simulink model "Observer_Luenberger_sensibilite_II_2023b"  (R2025a)
settings: Solver=FixedStepAuto  StartTime=0.0  StopTime=Inf  FixedStep=sub_step_size  RelTol=1e-3
PostLoadFcn:
  | , if any(exist('dsrtsu_mdlpostloadfcn', 'file') ~= 0), dsrtsu_mdlpostloadfcn('Execute', bdroot); end,
InitFcn:
  | , if any(exist('rtifpga_mdlclblib', 'file') ~= 0), rtifpga_mdlclblib('Init', bdroot); end,
values from neighbouring files (symbols this model uses):
  grandeurs_modales = load('grandeurs_modales.mat').MODAL    [varDQ_Observateur.m]
  k = 6    [varDQ_Observateur.m]
  mode_init = 1    [varDQ_Observateur.m]
  nb_plaques = numel(grandeurs_modales.n_modes)    [varDQ_Observateur.m]
  plaque_init = 1    [varDQ_Observateur.m]
  step_size = 1/frequency    (= 1.25e-06)    [varDQ_Observateur.m]
  V = 80    [varDQ_Observateur.m]
undefined symbols (not defined in the file or in its folder): conf, DiscIntNeverNeededParam
libraries: simulink x5, eeGeneralControl x2, slpidlib x1
Description:
  | Standard RTI1202 template.
  | Supported MATLAB version:  R2021a.
settings Model: Tag=RTI1202  DSRTSU_INTERNAL_RTI_VER=610  DSRTSU_INTERNAL_RTI_TYPE=rti1202  RTICANMMDATA=struct('GeneralSetupData',struct('modelroot','C:\Users\VM-User\Desktop\MigrationScripts','generalsettings',struct('filesettings',struct('destfolder',struct('Name','RTICANMM_FILES','Check',1),'buildfolder',struct('Name','.','Check',1),'AbsDestfolder',struct('Name','C:\Users\VM-User\Desktop\MigrationScripts\RTICANMM_FILES'),'AbsBuildfolder',struct('Name','C:\Users\VM-User\Desktop\MigrationScripts'))),'options',struct('addpaths',1,'rmpaths',1,'addtrcexclusion',true,'cannavigator',struct('checkmonitoring',0),'show_usrtrc',0,'use_usrtrc',0),'advanced',struct('options',ones(1,100)),'MPSetup',{{}},'RTI',struct('Type','RTI1202','Ver','7.17','Date','02-Nov-2021'),'modelname','','block','untitled'))  DSRTSU_INTERNAL_RTIFPGA=200  DSRTSU_INTERNAL_RTISTBM_VER=22.2  Creator=g.eymard  LastModifiedBy=user
settings SolverCC: AlgebraicLoopSolver=TrustRegion
settings DataIOCC: ReturnWorkspaceOutputs=off
settings OptimizationCC: BlockReduction=off  OptimizeBlockIOStorage=off  BufferReuse=off  GlobalBufferReuse=off  ExpressionFolding=off  LocalBlockOutputs=off  OptimizeDataStoreBuffers=off  BusAssignmentInplaceUpdate=off
settings DebuggingCC: UnconnectedInputMsg=warning  UnconnectedOutputMsg=warning  UnconnectedLineMsg=warning  PregeneratedLibrarySubsystemCodeDiagnostic=none  ArithmeticOperatorsInVariantConditions=warning
settings HardwareCC: ProdBitPerPointer=32.0  ProdBitPerSizeT=32.0  ProdBitPerPtrDiffT=32.0  ProdLargestAtomicInteger=Integer  ProdEndianess=BigEndian  ProdWordSize=32.0  ProdLongLongMode=on  ProdHWDeviceType=Custom Processor->Custom  TargetIntDivRoundTo=Zero  TargetEndianess=BigEndian  TargetHWDeviceType=Custom Processor->Custom
settings ModelReferenceCC: EnableRefExpFcnMdlSchedulingChecks=on  EnableParallelModelReferenceBuilds=on  ParallelModelReferenceMATLABWorkerInit=Load Top Model
settings SFSimCC: SimUseLocalCustomCode=off  MATLABDynamicMemAlloc=off  CustomCodeUndefinedFunction=UseInterfaceOnly
settings RTWCC: SystemTargetFile=rti1202.tlc  MakeCommand=make_rti  TemplateMakefile=rti1202.tmf  RTWUseLocalCustomCode=off  GPUComputeCapability=3.5  DLArmComputeVersion=19.05  Description=dSPACE DS1202 Hardware Platform
settings CodeAppCC: StateflowObjectComments=on
settings STFCustomTargetCC: SystemTargetFile=rti1202.tlc  MultiwordLength=2048.0  DynamicStringBufferSize=256.0  ParMdlRefBuildCompliant=on  GRTInterface=off  TaskMode=Low jitter, low latency tasks  FSIValue=0  TRCIsOmitVdOn=off  NISValue=1  LoadApplNonUI=ON  TRCGenerateDerivatives=off  RTICfgSetVer=610.0  PlatformSelectionPopup=Platform Name  CCompilerOptimizationOptsPopup_=Default  TimeScaleFactor=1.0  BoardName=ds1202  CCompilerOptimizationOptsNonUI=USE_DEFAULT  ExecutionMode=real-time  BoardNameNonUI=ds1202  EnableRealTimeTesting=on  InitialSimState=RUN  AllowReservedHostServiceNums=off  ExecutionModeNonUI=RTSIM  LoadAfterBuild=on  NetworkClientNonUI=OPTION_DISABLED  EnableRealTimeTestingNonUI=ON  TimeScaleFactorNonUI=OPTION_DISABLED  LoadToFlash=off  VDFType=TRC  TRCGenerateVirtualBlocks=off  TRCOnlyGlobals=off  TaskModeNonUI=LOW_JITTER  AssertionMode=OFF  TRCGenerateParamValues=off  TRCGenerateLabels=off  TRCGenerateStates=off
settings GRTTargetCC: TargetLangStandard=C89/C90 (ANSI)  CompOptLevelCompliant=off  ConcurrentExecutionCompliant=off  CombineOutputUpdateFcns=off  MatFileLogging=off  CPPClassGenCompliant=off  UseToolchainInfoCompliant=off
settings ConfigComp: CovMetricSettings=dswe

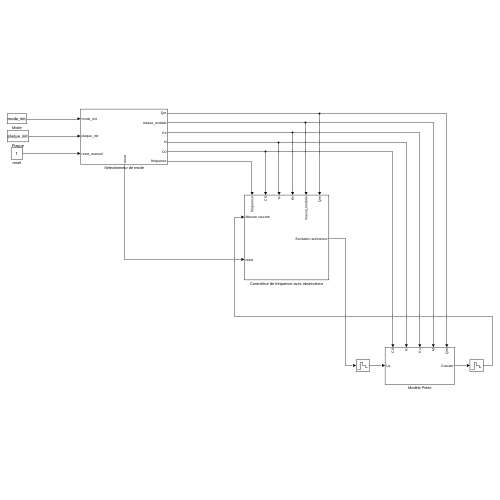
[thumbnail: Simulink's stored preview of the top-level diagram]
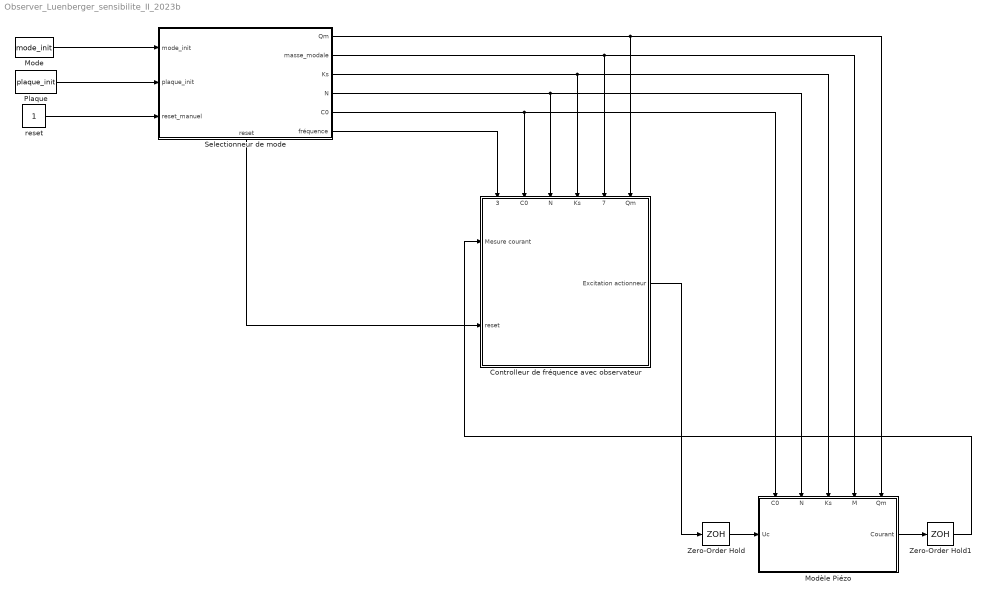
== system Observer_Luenberger_sensibilite_II_2023b ==
  Controlleur de fréquence avec observateur : Subsystem
      settings: PortSchema="{\"entries\":[{\"content\":{\"sides\":[{\"content\":{\"connectorIds\":[\"In1\",\"In2\"]},\"type\":\"ConnectorPlacement.EquallySpacedRectSide\",\"uuid\":\"530a0f3e-ee2a-4c6d-8269-1953a5690c3e\"},{\"content\":{\"connectorIds\":[\"Out1\"],\"side\":\"RIGHT\"},\"type\":\"ConnectorPlacement.EquallySpacedRectSide\",\"uuid\":\"d68bd64f-59c0-41d5-a325-75bb2cb6ca14\"},{\"content\":{\"connectorIds\":[\"In3\",\"In4\",\"In5\",\"In6\",\"In7\",\"In8\"],\"side\":\"TOP\"},\"type\":\"ConnectorPlacement.EquallySpacedRectSide\",\"uuid\":\"5a147631-f81e-4841-8249-4b54ec8a3c6f\"}]},\"type\":\"ConnectorPlacement.EquallySpacedConnector\",\"uuid\":\"7e21fd24-4eb3-483e-b19b-d5a2d9cc9389\"}],\"packageUris\":[\"http://schema.mathworks.com/mf0/Connector/R2020b\"],\"version\":\"1.0\"}"
  Mode : Constant  Value=mode_init  SampleTime=step_size
  Modèle Piézo : Subsystem
      settings: PortSchema="{\"entries\":[{\"content\":{\"sides\":[{\"content\":{\"connectorIds\":[\"In1\"]},\"type\":\"ConnectorPlacement.EquallySpacedRectSide\",\"uuid\":\"faf53970-2953-4ceb-88b4-68bddd4a0fc8\"},{\"content\":{\"connectorIds\":[\"Out1\"],\"side\":\"RIGHT\"},\"type\":\"ConnectorPlacement.EquallySpacedRectSide\",\"uuid\":\"a2d81363-6c92-409a-946a-c9fbc60f8e0e\"},{\"content\":{\"connectorIds\":[\"In2\",\"In3\",\"In4\",\"In5\",\"In6\"],\"side\":\"TOP\"},\"type\":\"ConnectorPlacement.EquallySpacedRectSide\",\"uuid\":\"99e0e8a0-eb56-42eb-b6d4-0f3431f01427\"}]},\"type\":\"ConnectorPlacement.EquallySpacedConnector\",\"uuid\":\"f1fccc4c-7076-4c73-816a-62f4c7feacf8\"}],\"packageUris\":[\"http://schema.mathworks.com/mf0/Connector/R2020b\"],\"version\":\"1.0\"}"
  Plaque : Constant  Value=plaque_init  SampleTime=step_size
  Selectionneur de mode : Subsystem
      settings: PortSchema="{\"entries\":[{\"content\":{\"sides\":[{\"content\":{\"connectorIds\":[\"In1\",\"In2\",\"In3\"]},\"type\":\"ConnectorPlacement.EquallySpacedRectSide\",\"uuid\":\"d44dafbb-4531-4740-8f88-9444e013c349\"},{\"content\":{\"connectorIds\":[\"Out1\",\"Out2\",\"Out3\",\"Out4\",\"Out5\",\"Out6\"],\"side\":\"RIGHT\"},\"type\":\"ConnectorPlacement.EquallySpacedRectSide\",\"uuid\":\"a0382d4c-1f36-46aa-81e2-f668b2a7eaab\"},{\"content\":{\"side\":\"TOP\"},\"type\":\"ConnectorPlacement.EquallySpacedRectSide\",\"uuid\":\"83c5ddd4-1965-4675-8f4e-255b2976aa40\"},{\"content\":{\"connectorIds\":[\"Out7\"],\"side\":\"BOTTOM\"},\"type\":\"ConnectorPlacement.EquallySpacedRectSide\",\"uuid\":\"40dab04f-efa3-4035-a07f-cd814a6077f4\"}]},\"type\":\"ConnectorPlacement.EquallySpacedConnector\",\"uuid\":\"ca871b34-0c20-4adb-897c-f336d60f682d\"}],\"packageUris\":[\"http://schema.mathworks.com/mf0/Connector/R2020b\"],\"version\":\"1.0\"}"
  Zero-Order Hold : ZeroOrderHold  SampleTime=step_size
  Zero-Order Hold1 : ZeroOrderHold  SampleTime=step_size
  reset : Constant  SampleTime=step_size
  wires:
  Mode/1 -> Selectionneur de mode/1(mode_init)
  Plaque/1 -> Selectionneur de mode/2(plaque_init)
  reset/1 -> Selectionneur de mode/3(reset_manuel)
  Selectionneur de mode/7(reset) -> Controlleur de fréquence avec observateur/2(reset)
  Selectionneur de mode/6(fréquence) -> Controlleur de fréquence avec observateur/3(fréquence)
  Selectionneur de mode/5(C0) -> Modèle Piézo/2(C0), Controlleur de fréquence avec observateur/4(C0)
  Selectionneur de mode/2(masse_modale) -> Modèle Piézo/5(M), Controlleur de fréquence avec observateur/7(masse_modale)
  Selectionneur de mode/4(N) -> Modèle Piézo/3(N), Controlleur de fréquence avec observateur/5(N)
  Selectionneur de mode/3(Ks) -> Modèle Piézo/4(Ks), Controlleur de fréquence avec observateur/6(Ks)
  Controlleur de fréquence avec observateur/1(Excitation actionneur) -> Zero-Order Hold/1
  Modèle Piézo/1(Courant) -> Zero-Order Hold1/1
  Zero-Order Hold/1 -> Modèle Piézo/1(Uc)
  Zero-Order Hold1/1 -> Controlleur de fréquence avec observateur/1(Mesure courant)
  Selectionneur de mode/1(Qm) -> Modèle Piézo/6(Qm), Controlleur de fréquence avec observateur/8(Qm)

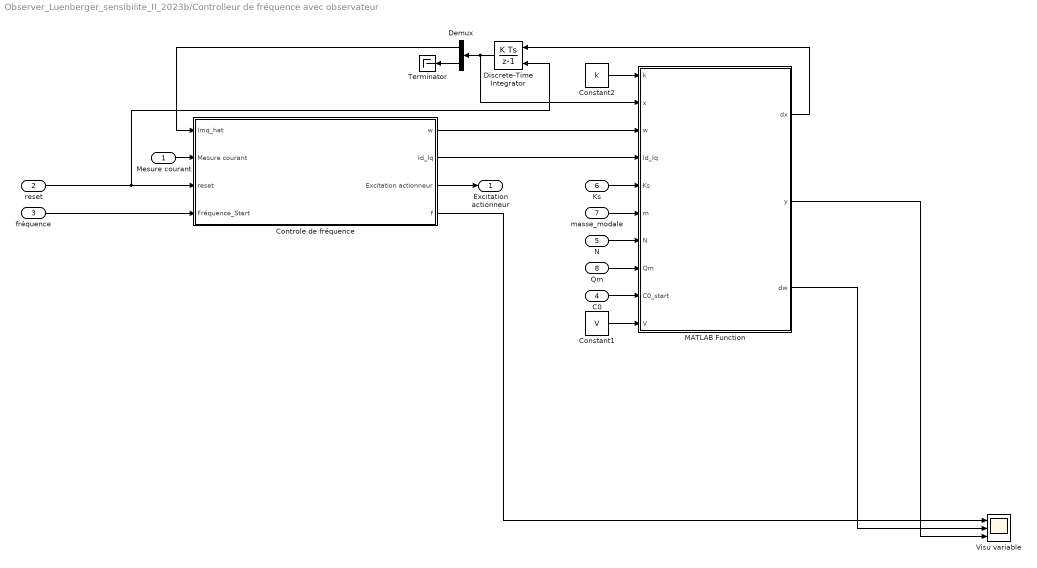
== system Observer_Luenberger_sensibilite_II_2023b/Controlleur de fréquence avec observateur ==
  Mesure courant : Inport
  reset : Inport  Port=2
  fréquence : Inport  Port=3
  C0 : Inport  Port=4
  N : Inport  Port=5
  Ks : Inport  Port=6
  masse_modale : Inport  Port=7
  Qm : Inport  Port=8
  Constant1 : Constant  Value=V  SampleTime=step_size
  Constant2 : Constant  Value=k  SampleTime=step_size
  Controle de fréquence : Subsystem
  Demux : Demux  Outputs=2
  Discrete-Time Integrator : DiscreteIntegrator  ExternalReset=rising  InitialCondition=[0; 0]  SampleTime=-1  ICPrevOutput=DiscIntNeverNeededParam  ICPrevScaledInput=DiscIntNeverNeededParam
  MATLAB Function : MATLAB Function  TreatAsAtomicUnit=on
  Terminator : Terminator
  Visu variable : Scope  NumInputPorts=3
      settings: ActiveDisplayYMinimum=-632.5898  ActiveDisplayYMaximum=4274.0061
  Excitation actionneur : Outport
  wires:
  Controle de fréquence/2(Id_Iq) -> MATLAB Function/4(Id_Iq)
  Discrete-Time Integrator/1 -> MATLAB Function/2(x), Demux/1
  Mesure courant/1 -> Controle de fréquence/2(Mesure courant)
  Controle de fréquence/1(w) -> MATLAB Function/3(w)
  Controle de fréquence/3(Excitation actionneur) -> Excitation actionneur/1
  MATLAB Function/1(dx) -> Discrete-Time Integrator/1
  Demux/1 -> Controle de fréquence/1(Imq_hat)
  Controle de fréquence/4(f) -> Visu variable/1
  MATLAB Function/3(dw) -> Visu variable/2
  MATLAB Function/2(y) -> Visu variable/3
  reset/1 -> Discrete-Time Integrator/2, Controle de fréquence/3(reset)
  Demux/2 -> Terminator/1
  fréquence/1 -> Controle de fréquence/4(Fréquence_Start)
  masse_modale/1 -> MATLAB Function/6(m)
  Ks/1 -> MATLAB Function/5(Ks)
  N/1 -> MATLAB Function/7(N)
  Constant1/1 -> MATLAB Function/10(V)
  C0/1 -> MATLAB Function/9(C0_start)
  Qm/1 -> MATLAB Function/8(Qm)
  Constant2/1 -> MATLAB Function/1(k)

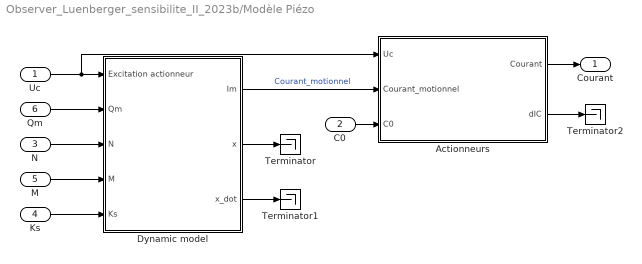
== system Observer_Luenberger_sensibilite_II_2023b/Modèle Piézo ==
  Uc : Inport
  C0 : Inport  Port=2
  N : Inport  Port=3
  Ks : Inport  Port=4
  M : Inport  Port=5
  Qm : Inport  Port=6
  Actionneurs : Subsystem
  Dynamic model : Subsystem
  Terminator : Terminator
  Terminator1 : Terminator
  Terminator2 : Terminator
  Courant : Outport
  wires:
  Actionneurs/2(dIC) -> Terminator2/1
  Dynamic model/3(x_dot) -> Terminator1/1
  Dynamic model/2(x) -> Terminator/1
  Dynamic model/1(Im) -> Actionneurs/2(Courant_motionnel)  "Courant_motionnel"
  M/1 -> Dynamic model/4(M)
  N/1 -> Dynamic model/3(N)
  Ks/1 -> Dynamic model/5(Ks)
  Uc/1 -> Actionneurs/1(Uc), Dynamic model/1(Excitation actionneur)
  Actionneurs/1(Courant) -> Courant/1
  C0/1 -> Actionneurs/3(C0)
  Qm/1 -> Dynamic model/2(Qm)

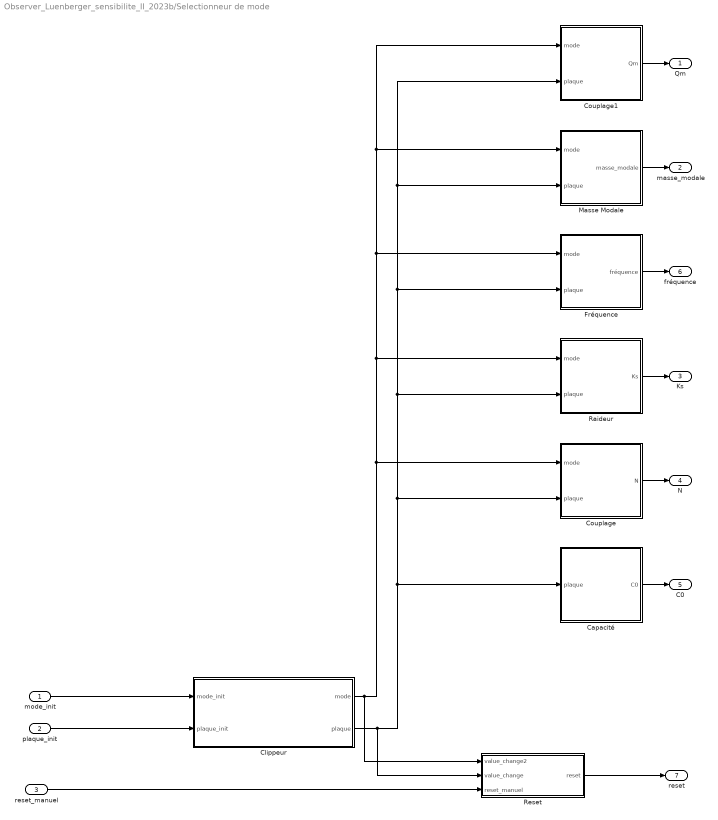
== system Observer_Luenberger_sensibilite_II_2023b/Selectionneur de mode ==
  mode_init : Inport
  plaque_init : Inport  Port=2
  reset_manuel : Inport  Port=3
  Capacité : Subsystem
  Clippeur : Subsystem
  Couplage : Subsystem
  Couplage1 : Subsystem
  Fréquence : Subsystem
  Masse Modale : Subsystem
  Raideur : Subsystem
  Reset : Subsystem
  Qm : Outport
  masse_modale : Outport  Port=2
  Ks : Outport  Port=3
  N : Outport  Port=4
  C0 : Outport  Port=5
  fréquence : Outport  Port=6
  reset : Outport  Port=7
  wires:
  mode_init/1 -> Clippeur/1(mode_init)
  Masse Modale/1(masse_modale) -> masse_modale/1
  Reset/1(reset) -> reset/1
  plaque_init/1 -> Clippeur/2(plaque_init)
  Fréquence/1(fréquence) -> fréquence/1
  reset_manuel/1 -> Reset/3(reset_manuel)
  Raideur/1(Ks) -> Ks/1
  Couplage/1(N) -> N/1
  Capacité/1(C0) -> C0/1
  Clippeur/1(mode) -> Reset/1(value_change2), Couplage/1(mode), Fréquence/1(mode), Couplage1/1(mode), Masse Modale/1(mode), Raideur/1(mode)
  Clippeur/2(plaque) -> Reset/2(value_change), Capacité/1(plaque), Couplage/2(plaque), Fréquence/2(plaque), Couplage1/2(plaque), Masse Modale/2(plaque), Raideur/2(plaque)
  Couplage1/1(Qm) -> Qm/1

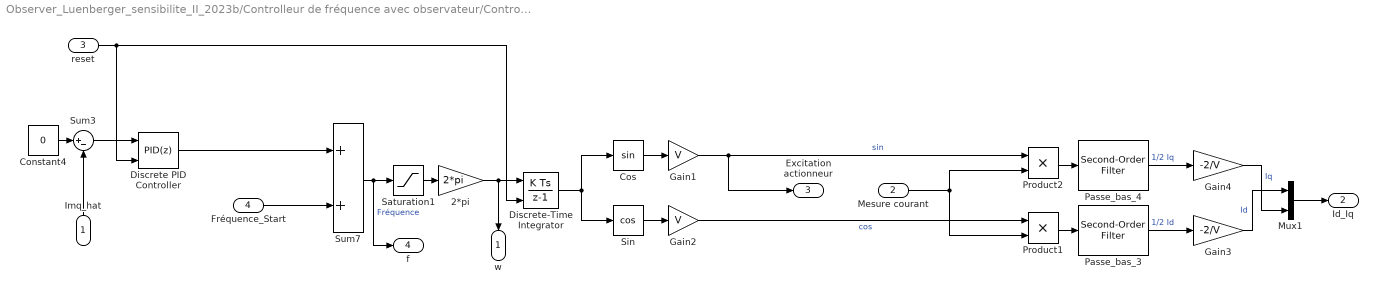
== system Observer_Luenberger_sensibilite_II_2023b/Controlleur de fréquence avec observateur/Controle de fréquence ==
  Imq_hat : Inport
  Mesure courant : Inport  Port=2
  reset : Inport  Port=3
  Fréquence_Start : Inport  Port=4
  " Mux1" : Mux  Inputs=2
  2*pi : Gain  Gain=2*pi
  Constant4 : Constant  Value=0  SampleTime=step_size
  Cos : Trigonometry
  Discrete PID Controller : slpidlib/PID Controller  Controller=PID  Form=Parallel  TimeDomain=Discrete-time  UseExternalTs=off  SampleTime=step_size  IntegratorMethod=Forward Euler  FilterMethod=Forward Euler  ControllerParametersSource=internal  P=-10000  I=-9e6/2  UseKiTs=off  D=0  UseExternalDerivativeSource=off  N=100  UseFilter=on  TunerSelectOption=Transfer Function Based (PID Tuner App)  InitialConditionSource=internal  InitialConditionForIntegrator=0  InitialConditionForFilter=0  DifferentiatorICPrevScaledInput=0  ExternalReset=rising  TrackingMode=off  Kt=1  LimitOutput=off  SatLimitsSource=internal  UpperSaturationLimit=inf  LowerSaturationLimit=-inf  LinearizeAsGain=off  AntiWindupMode=none  Kb=1  LimitIntegrator=off  UpperIntegratorSaturationLimit=inf  LowerIntegratorSaturationLimit=-inf  POutMin=[]  POutMax=[]  IOutMin=[]  IOutMax=[]  DOutMin=[]  DOutMax=[]  NOutMin=[]  NOutMax=[]  SumOutMin=[]  SumOutMax=[]  SaturationOutMin=[]  SaturationOutMax=[]  PParamMin=[]  PParamMax=[]  IParamMin=[]  IParamMax=[]  DParamMin=[]  DParamMax=[]  NParamMin=[]  NParamMax=[]  KbParamMin=[]  KbParamMax=[]  KtParamMin=[]  KtParamMax=[]  KbOutMin=[]  KbOutMax=[]  KtOutMin=[]  KtOutMax=[]  IntegratorOutMin=[]  IntegratorOutMax=[]  FilterOutMin=[]  FilterOutMax=[]  SumI1OutMin=[]  SumI1OutMax=[]  SumI2OutMin=[]  SumI2OutMax=[]  SumI3OutMin=[]  SumI3OutMax=[]  SumI4OutMin=[]  SumI4OutMax=[]  SumDOutMin=[]  SumDOutMax=[]  DifferentiatorOutMin=[]  DifferentiatorOutMax=[]  FilterDiffOutCoefMin=[]  FilterDiffOutCoefMax=[]  ReciprocalOutMin=[]  ReciprocalOutMax=[]  SumDenOutMin=[]  SumDenOutMax=[]  SumNumOutMin=[]  SumNumOutMax=[]  DivideOutMin=[]  DivideOutMax=[]  UdiffTsProdOutMin=[]  UdiffTsProdOutMax=[]  NTsProdOutMin=[]  NTsProdOutMax=[]  UintegralTsProdOutMin=[]  UintegralTsProdOutMax=[]  UngainTsProdOutMin=[]  UngainTsProdOutMax=[]  ClampingZeroOutDataTypeStr=Inherit: Inherit via back propagation  ClampingZeroOutMin=[]  ClampingZeroOutMax=[]  FilterDenConstantOutDataTypeStr=Inherit: Inherit via back propagation  FilterDenConstantOutMin=[]  FilterDenConstantOutMax=[]  PCopyOutDataTypeStr=Inherit: Inherit via back propagation  PCopyOutMin=[]  PCopyOutMax=[]  NCopyOutDataTypeStr=Inherit: Inherit via back propagation  NCopyOutMin=[]  NCopyOutMax=[]  IntegratorContinuousStateAttributes=''  IntegratorStateMustResolveToSignalObject=off  IntegratorRTWStateStorageClass=Auto  FilterContinuousStateAttributes=''  FilterStateMustResolveToSignalObject=off  FilterRTWStateStorageClass=Auto  ParallelPVariant=InternalParameters  IdealPVariant=Disabled  IVariant=InternalParameters  DVariant=InternalParameters  IntegratorVariant=Discrete  SatVariant=Disabled  AWVariant=Passthrough  PCopyVariant=Disabled  TRVariant=Disabled  FdbkBlocksVariant=Forward  IdealPFdbkVariant=Disabled  SatFdbkVariant=Disabled  DerivativeFilterVariant=ForwardEulerFilter  NVariant=InternalParameters  NCopyVariant=Disabled  FilterICVariant=InternalICsFilter  IntegratorICVariant=InternalICs  ExternalResetVariant=ExternalReset  TRSumVariant=Passthrough  SumFdbkVariant=Disabled  SumVariant=Sum_PID  TsampFilterVariant=InternalTs  TsampNgainVariant=Passthrough  TsampIntegralVariant=Disabled_SignalSpec  ExternalSaturationOutDataTypeStr=Inherit: Same as second input  DerivativeSourceVariant=ErrorSignal  PreIntVariant=InternalPreInt
  Discrete-Time Integrator : DiscreteIntegrator  ExternalReset=rising  SampleTime=-1  ICPrevOutput=DiscIntNeverNeededParam  ICPrevScaledInput=DiscIntNeverNeededParam
  Gain1 : Gain  Gain=V
  Gain2 : Gain  Gain=V
  Gain3 : Gain  Gain=-2/V
  Gain4 : Gain  Gain=-2/V
  Passe_bas_3 : eeGeneralControl/Second-Order Filter  FilterType=Low-pass  fn=50  Zeta=0.707  Ts=-1  A0=1e-6  Ph0=0  f0=0  b0=0
  Passe_bas_4 : eeGeneralControl/Second-Order Filter  FilterType=Low-pass  fn=50  Zeta=0.707  Ts=-1  A0=1e-6  Ph0=0  f0=0  b0=0
  Product1 : Product
  Product2 : Product
  Saturation1 : Saturate  UpperLimit=inf  LowerLimit=0
  Sin : Trigonometry  Operator=cos
  Sum3 : Sum  Inputs=|+-
  Sum7 : Sum
  w : Outport
  Id_Iq : Outport  Port=2
  Excitation actionneur : Outport  Port=3
  f : Outport  Port=4
  wires:
  Cos/1 -> Gain1/1
  Fréquence_Start/1 -> Sum7/2
  Discrete-Time Integrator/1 -> Sin/1, Cos/1
  2*pi/1 -> Discrete-Time Integrator/1, w/1
  Sin/1 -> Gain2/1
  Discrete PID Controller/1 -> Sum7/1
  Constant4/1 -> Sum3/1
  Imq_hat/1 -> Sum3/2
  Sum3/1 -> Discrete PID Controller/1
  Gain2/1 -> Product1/1  "cos"
  Passe_bas_3/1 -> Gain3/1  "1/2 Id"
  Mesure courant/1 -> Product2/2, Product1/2
  Product2/1 -> Passe_bas_4/1
  Passe_bas_4/1 -> Gain4/1  "1/2 Iq"
  Product1/1 -> Passe_bas_3/1
  Gain1/1 -> Excitation actionneur/1, Product2/1  "sin"
  " Mux1"/1 -> Id_Iq/1
  Sum7/1 -> f/1, Saturation1/1  "Fréquence"
  Saturation1/1 -> 2*pi/1
  reset/1 -> Discrete-Time Integrator/2, Discrete PID Controller/2
  Gain4/1 -> " Mux1"/2  "Iq"
  Gain3/1 -> " Mux1"/1  "Id"

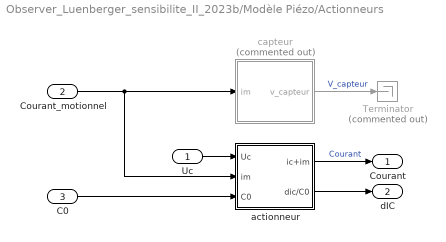
== system Observer_Luenberger_sensibilite_II_2023b/Modèle Piézo/Actionneurs ==
  Uc : Inport
  Courant_motionnel : Inport  Port=2
  C0 : Inport  Port=3
  Terminator : Terminator  Commented=on
  actionneur : Subsystem
  capteur : Subsystem  Commented=on
  Courant : Outport
  dIC : Outport  Port=2
  wires:
  actionneur/1(ic+im) -> Courant/1  "Courant"
  Uc/1 -> actionneur/1(Uc)
  capteur/1(v_capteur) -> Terminator/1  "V_capteur"
  Courant_motionnel/1 -> capteur/1(im), actionneur/2(im)
  actionneur/2(dic/C0) -> dIC/1
  C0/1 -> actionneur/3(C0)

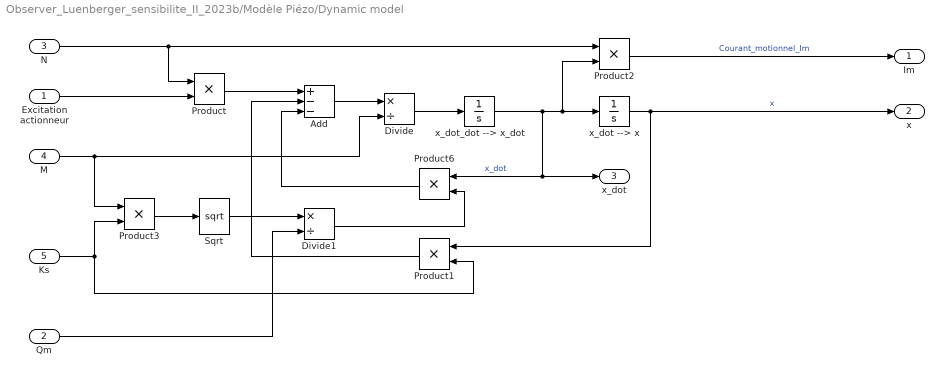
== system Observer_Luenberger_sensibilite_II_2023b/Modèle Piézo/Dynamic model ==
  Excitation actionneur : Inport
  Qm : Inport  Port=2
  N : Inport  Port=3
  M : Inport  Port=4
  Ks : Inport  Port=5
  Add : Sum  Inputs=+--
  Divide : Product  Inputs=*/
  Divide1 : Product  Inputs=*/
  Product{,1..3,6} (5 alike) : Product
  Sqrt : Sqrt
  x_dot --> x : Integrator
  x_dot_dot --> x_dot : Integrator
  Im : Outport
  x : Outport  Port=2
  x_dot : Outport  Port=3
  wires:
  M/1 -> Divide/2, Product3/1
  N/1 -> Product/1, Product2/1
  x_dot_dot --> x_dot/1 -> Product2/2, x_dot --> x/1, x_dot/1, Product6/1  "x_dot"
  Ks/1 -> Product1/2, Product3/2
  Product1/1 -> Add/2
  Divide1/1 -> Product6/2
  Product6/1 -> Add/3
  x_dot --> x/1 -> x/1, Product1/1  "x"
  Add/1 -> Divide/1
  Product3/1 -> Sqrt/1
  Product/1 -> Add/1
  Excitation actionneur/1 -> Product/2
  Divide/1 -> x_dot_dot --> x_dot/1
  Product2/1 -> Im/1  "Courant_motionnel_Im"
  Sqrt/1 -> Divide1/1
  Qm/1 -> Divide1/2

== system Observer_Luenberger_sensibilite_II_2023b/Selectionneur de mode/Capacité ==
  plaque : Inport
  Constant1 : Constant  Value=grandeurs_modales.C0  SampleTime=step_size
  Selector : Selector  InputPortWidth=nb_plaques  IndexOptions=Index vector (port)  Indices=[1 3]  OutputSizes=1
  C0 : Outport
  wires:
  Constant1/1 -> Selector/1
  Selector/1 -> C0/1
  plaque/1 -> Selector/2

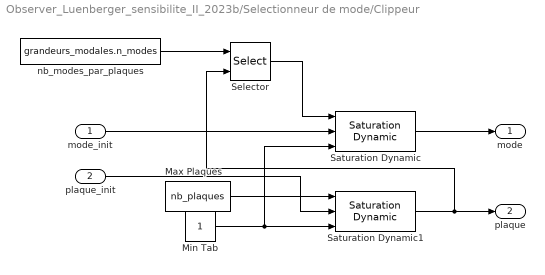
== system Observer_Luenberger_sensibilite_II_2023b/Selectionneur de mode/Clippeur ==
  mode_init : Inport
  plaque_init : Inport  Port=2
  Max Plaques : Constant  Value=nb_plaques  SampleTime=step_size
  Min Tab : Constant  SampleTime=step_size
  Saturation Dynamic : simulink/Discontinuities/Saturation Dynamic  OutMin=[]  OutMax=[]  OutDataTypeStr=Inherit: Same as second input  OutDataType=fixdt(1, 16)  OutScaling=2^-10  DoSatur=off
  Saturation Dynamic1 : simulink/Discontinuities/Saturation Dynamic  OutMin=[]  OutMax=[]  OutDataTypeStr=Inherit: Same as second input  OutDataType=fixdt(1, 16)  OutScaling=2^-10  DoSatur=off
  Selector : Selector  InputPortWidth=nb_plaques  IndexOptions=Index vector (port)  Indices=[1 3]  OutputSizes=1
  nb_modes_par_plaques : Constant  Value=grandeurs_modales.n_modes  SampleTime=step_size
  mode : Outport
  plaque : Outport  Port=2
  wires:
  Min Tab/1 -> Saturation Dynamic/3, Saturation Dynamic1/3
  Saturation Dynamic1/1 -> plaque/1, Selector/2
  plaque_init/1 -> Saturation Dynamic1/2
  Max Plaques/1 -> Saturation Dynamic1/1
  nb_modes_par_plaques/1 -> Selector/1
  Saturation Dynamic/1 -> mode/1
  Selector/1 -> Saturation Dynamic/1
  mode_init/1 -> Saturation Dynamic/2

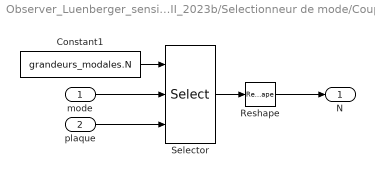
== system Observer_Luenberger_sensibilite_II_2023b/Selectionneur de mode/Couplage ==
  mode : Inport
  plaque : Inport  Port=2
  Constant1 : Constant  Value=grandeurs_modales.N  SampleTime=step_size
  Reshape : Reshape  OutputDimensionality=Customize  OutputDimensions=1
  Selector : Selector  NumberOfDimensions=2  InputPortWidth=3  IndexOptions=Index vector (port),Index vector (port)  Indices=[1 3],1  OutputSizes=1,1
  N : Outport
  wires:
  Constant1/1 -> Selector/1
  mode/1 -> Selector/2
  Selector/1 -> Reshape/1
  plaque/1 -> Selector/3
  Reshape/1 -> N/1

== system Observer_Luenberger_sensibilite_II_2023b/Selectionneur de mode/Couplage1 ==
  mode : Inport
  plaque : Inport  Port=2
  Constant1 : Constant  Value=grandeurs_modales.Qm  SampleTime=step_size
  Reshape : Reshape  OutputDimensionality=Customize  OutputDimensions=1
  Selector : Selector  NumberOfDimensions=2  InputPortWidth=3  IndexOptions=Index vector (port),Index vector (port)  Indices=[1 3],1  OutputSizes=1,1
  Qm : Outport
  wires:
  Constant1/1 -> Selector/1
  mode/1 -> Selector/2
  Selector/1 -> Reshape/1
  plaque/1 -> Selector/3
  Reshape/1 -> Qm/1

== system Observer_Luenberger_sensibilite_II_2023b/Selectionneur de mode/Fréquence ==
  mode : Inport
  plaque : Inport  Port=2
  Constant1 : Constant  Value=grandeurs_modales.f  SampleTime=step_size
  Reshape : Reshape  OutputDimensionality=Customize  OutputDimensions=1
  Selector : Selector  NumberOfDimensions=2  InputPortWidth=3  IndexOptions=Index vector (port),Index vector (port)  Indices=[1 3],1  OutputSizes=1,1
  fréquence : Outport
  wires:
  Constant1/1 -> Selector/1
  mode/1 -> Selector/2
  Selector/1 -> Reshape/1
  plaque/1 -> Selector/3
  Reshape/1 -> fréquence/1

== system Observer_Luenberger_sensibilite_II_2023b/Selectionneur de mode/Masse Modale ==
  mode : Inport
  plaque : Inport  Port=2
  Constant1 : Constant  Value=grandeurs_modales.M  SampleTime=step_size
  Reshape : Reshape  OutputDimensionality=Customize  OutputDimensions=1
  Selector : Selector  NumberOfDimensions=2  InputPortWidth=3  IndexOptions=Index vector (port),Index vector (port)  Indices=[1 3],1  OutputSizes=1,1
  masse_modale : Outport
  wires:
  Constant1/1 -> Selector/1
  mode/1 -> Selector/2
  plaque/1 -> Selector/3
  Selector/1 -> Reshape/1
  Reshape/1 -> masse_modale/1

== system Observer_Luenberger_sensibilite_II_2023b/Selectionneur de mode/Raideur ==
  mode : Inport
  plaque : Inport  Port=2
  Constant1 : Constant  Value=grandeurs_modales.Ks  SampleTime=step_size
  Reshape : Reshape  OutputDimensionality=Customize  OutputDimensions=1
  Selector : Selector  NumberOfDimensions=2  InputPortWidth=3  IndexOptions=Index vector (port),Index vector (port)  Indices=[1 3],1  OutputSizes=1,1
  Ks : Outport
  wires:
  Constant1/1 -> Selector/1
  mode/1 -> Selector/2
  Selector/1 -> Reshape/1
  plaque/1 -> Selector/3
  Reshape/1 -> Ks/1

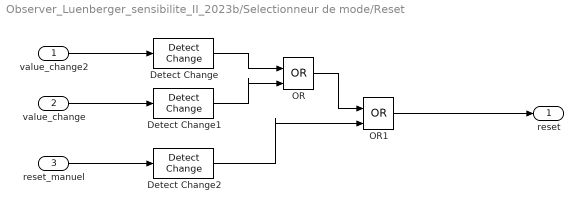
== system Observer_Luenberger_sensibilite_II_2023b/Selectionneur de mode/Reset ==
  value_change2 : Inport
  value_change : Inport  Port=2
  reset_manuel : Inport  Port=3
  Detect Change : simulink/Logic and Bit Operations/Detect Change  vinit=0  OutDataTypeStr=boolean
  Detect Change1 : simulink/Logic and Bit Operations/Detect Change  vinit=0  OutDataTypeStr=boolean
  Detect Change2 : simulink/Logic and Bit Operations/Detect Change  vinit=0  OutDataTypeStr=boolean
  OR : Logic  Operator=OR  IconShape=distinctive  AllPortsSameDT=off  OutDataTypeStr=boolean
  OR1 : Logic  Operator=OR  IconShape=distinctive  AllPortsSameDT=off  OutDataTypeStr=boolean
  reset : Outport
  wires:
  OR1/1 -> reset/1
  Detect Change1/1 -> OR/2
  OR/1 -> OR1/1
  reset_manuel/1 -> Detect Change2/1
  Detect Change/1 -> OR/1
  Detect Change2/1 -> OR1/2
  value_change/1 -> Detect Change1/1
  value_change2/1 -> Detect Change/1

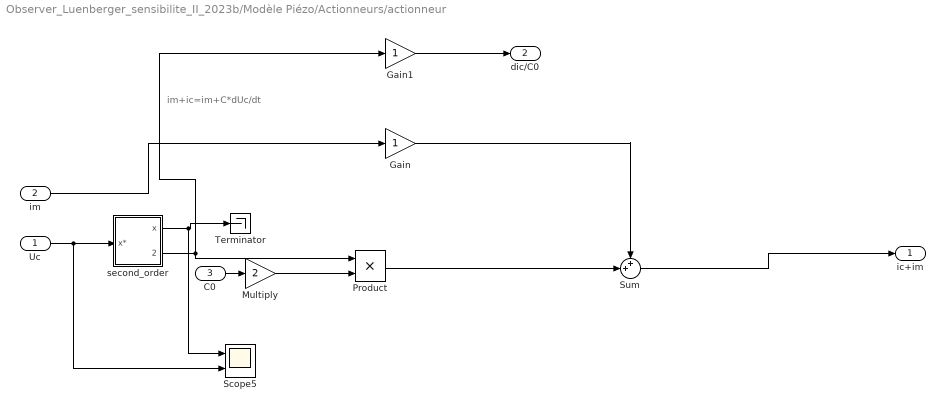
== system Observer_Luenberger_sensibilite_II_2023b/Modèle Piézo/Actionneurs/actionneur ==
  note: im+ic=im+C*dUc/dt
  Uc : Inport
  im : Inport  Port=2
  C0 : Inport  Port=3
  Gain : Gain
  Gain1 : Gain
  Multiply : Gain  Gain=2
  Product : Product
  Scope5 : Scope  NumInputPorts=2
      settings: ActiveDisplayYMinimum=-35.929000784188318  ActiveDisplayYMaximum=42.033035268061695  DataLoggingVariableName=ScopeData5
  Sum : Sum  Inputs=++|
  Terminator : Terminator
  second_order : Subsystem  mask{w=2*pi*50000, m=1}
      mask prompts: w "Pulsation propre"; m "Amortissement"
  ic+im : Outport
  dic/C0 : Outport  Port=2
  wires:
  im/1 -> Gain/1
  Product/1 -> Sum/2
  Sum/1 -> ic+im/1
  Uc/1 -> Scope5/2, second_order/1(x*)
  second_order/2(dx_dt) -> Product/1, Gain1/1
  second_order/1(x) -> Scope5/1, Terminator/1
  Gain/1 -> Sum/1
  Gain1/1 -> dic/C0/1
  Multiply/1 -> Product/2
  C0/1 -> Multiply/1

== system Observer_Luenberger_sensibilite_II_2023b/Modèle Piézo/Actionneurs/capteur ==
  im : Inport
  Add1 : Sum  Inputs=-+
  Gain1 : Gain  Gain=1/conf.det.Ccapt
  Gain2 : Gain  Gain=1/conf.det.Rcapt
  Integrator2 : Integrator
  v_capteur : Outport
  wires:
  Gain2/1 -> Add1/1
  Add1/1 -> Gain1/1
  Gain1/1 -> Integrator2/1  "duc/dt"
  Integrator2/1 -> v_capteur/1, Gain2/1  "v_capteur"
  im/1 -> Add1/2

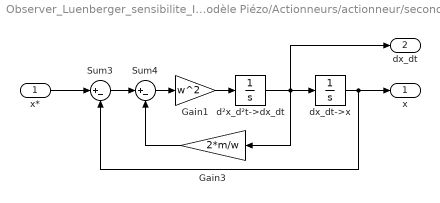
== system Observer_Luenberger_sensibilite_II_2023b/Modèle Piézo/Actionneurs/actionneur/second_order ==
  x* : Inport
  Gain1 : Gain  Gain=w^2
  Gain3 : Gain  Gain=2*m/w
  Sum3 : Sum  Inputs=|+-
  Sum4 : Sum  Inputs=|+-
  dx_dt->x : Integrator
  d²x_d²t->dx_dt : Integrator
  x : Outport
  dx_dt : Outport  Port=2
  wires:
  Sum3/1 -> Sum4/1
  Gain1/1 -> d²x_d²t->dx_dt/1
  d²x_d²t->dx_dt/1 -> dx_dt/1, Gain3/1, dx_dt->x/1
  Sum4/1 -> Gain1/1
  Gain3/1 -> Sum4/2
  x*/1 -> Sum3/1
  dx_dt->x/1 -> x/1, Sum3/2

== matlab function Observer_Luenberger_sensibilite_II_2023b/Controlleur de fréquence avec observateur/MATLAB Function ==
  data: k input; dx output; x input; y output; w input; Id_Iq input; Ks input; m input; N input; Qm input; C0_start input; V input; dw output
function [dx, y, dw] = Luenberger_obs_sensi_multi(k, x, w, Id_Iq, Ks, m, N, Qm, C0_start, V)

    % --- Constantes système ---
    w0 = sqrt(Ks/m);
    C0 = C0_start*2;
    A  = [-w0/(2*Qm), 0; 0, -w0/(2*Qm)];
    B  = [0; -N^2/(2*m)];
    dw = k * (w - w0); 
    Atotal = A + [0, dw; -dw, 0];
    D = [0; C0*w];
    Cmat = eye(2);

    l = (k-1)*(w0/(2 * Qm));
    L = l * [1, 0; 0, 1];

    % --- Matrice boucle fermée ---
    % Acl = Atotal - L * Cmat;

    % --- DYNAMIQUE PRINCIPALE ---
    error = Id_Iq - (Cmat * x + D * V);
    dx = Atotal * x + B * V + L * error;

    % --- SORTIE ---
    y = Cmat * x + D * V;

    
    % % --- SENSIBILITÉS : zéro avant t_sensi ---
    % t_sensi = 0.02;
    % if t < t_sensi
    %     dsx_C0 = zeros(size(x));
    %     dsx_m  = zeros(size(x));
    %     dsx_Ks = zeros(size(x));
    %     dsy_C0 = zeros(size(y));
    %     dsy_m  = zeros(size(y));
    %     dsy_Ks = zeros(size(y));
    %     S_C0   = [0; 1.004];
    %     S_m    = zeros(size(y));
    %     S_Ks   = zeros(size(y));
    %     return
    % end
    % 
    % % --- SENSIBILITÉS (calcul normal) ---
    % 
    % % Dérivées partielles pour C0
    % dD_C0 = [0; w];
    % 
    % % Dérivées partielles pour m
    % dw0_dm = -w0 / (2*m);
    % dA_m = [-(dw0_dm)/(2*Qm), 0; 0, -(dw0_dm)/(2*Qm)];
    % dB_m = [0; -N^2/(2*m^2)];
    % dAtotal_m = dA_m + [0, -k*dw0_dm; k*dw0_dm, 0];
    % 
    % % Dérivées partielles pour Ks
    % dw0_dKs = 0.5 / (w0*m);
    % dA_Ks = [-(dw0_dKs)/(2*Qm), 0; 0, -(dw0_dKs)/(2*Qm)];
    % dAtotal_Ks = dA_Ks + [0, -k*dw0_dKs; k*dw0_dKs, 0];
    % 
    % % Propagation des sensibilités (boucle fermée)
    % dsx_C0 = Acl * sx_C0 - L * dD_C0 * u;
    % dsx_m  = Acl * sx_m  + dAtotal_m * x + dB_m * u;
    % dsx_Ks = Acl * sx_Ks + dAtotal_Ks * x;
    % 
    % % Sensibilités de la sortie
    % dsy_C0 = Cmat * sx_C0 + dD_C0 * u;
    % dsy_m  = Cmat * sx_m;
    % dsy_Ks = Cmat * sx_Ks;
    % 
    % % Normalisation
    % y_safe = y; y_safe(abs(y_safe) < 1e-12) = 1e-12;
    % S_C0 = (C0 ./ y_safe) .* dsy_C0;
    % S_m  = (m  ./ y_safe) .* dsy_m;
    % S_Ks = (Ks ./ y_safe) .* dsy_Ks;

end
